simulink model "sys_sim"  (R2025a)
settings: Solver=VariableStepAuto  StartTime=0.0  StopTime=50  RelTol=1e-3
values from neighbouring files (symbols this model uses):
  f = 0.0077* (pi/180)    (= 0.000134390352404)    [parameters.m]    (also in q12 0.1 sim.mat; q12 0.2 sim.mat; q12 0.3 sim.mat; q12 0.36 sim.mat)
  ng = 5.25    [parameters.m]    (also in q12 0.1 sim.mat; q12 0.2 sim.mat; q12 0.3 sim.mat; q12 0.36 sim.mat)
  Ra = 2.08    [parameters.m]    (also in q12 0.1 sim.mat; q12 0.2 sim.mat; q12 0.3 sim.mat; q12 0.36 sim.mat)
undefined symbols (not defined in the file or in its folder): j, Km
settings Model: Creator=ASUS  LastModifiedBy=ASUS

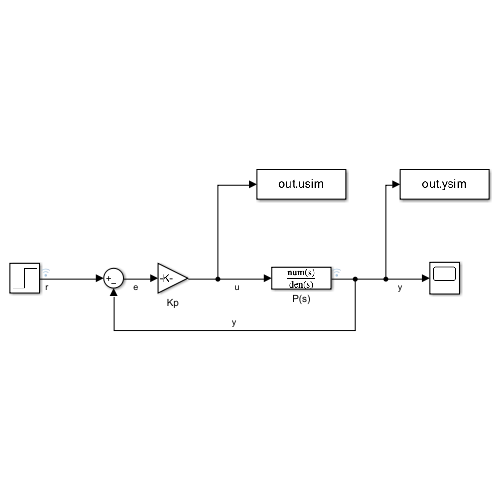
[thumbnail: Simulink's stored preview of the top-level diagram]
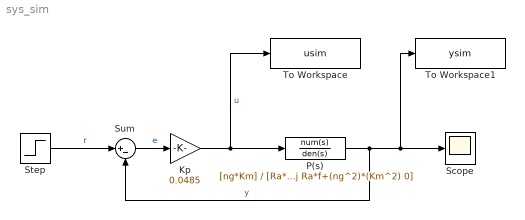
== system sys_sim ==
  Kp : Gain  Gain=0.0485
  P(s) : TransferFcn  Numerator=[ng*Km]  Denominator=[Ra*j Ra*f+(ng^2)*(Km^2) 0]
  Scope : Scope
      settings: ActiveDisplayYMinimum=-8156.1804750566789  ActiveDisplayYMaximum=11454.73502529323
  Step : Step  After=30  SampleTime=0
  Sum : Sum  Inputs=|+-
  To Workspace : ToWorkspace  VariableName=usim  SaveFormat=Timeseries  SampleTime=-1
  To Workspace1 : ToWorkspace  VariableName=ysim  SaveFormat=Timeseries  SampleTime=-1
  wires:
  Step/1 -> Sum/1  "r"
  Kp/1 -> To Workspace/1, P(s)/1  "u"
  P(s)/1 -> To Workspace1/1, Scope/1, Sum/2  "y"
  Sum/1 -> Kp/1  "e"
